simulink model "Ann_Pedals_SavePopup_newPwrCalib"  (Simulink 6.6)
settings: Solver=ode3  StartTime=0.0  StopTime=inf  RelTol=1e-3
StopFcn:
  | %% Name .mat file
  | 
  |     datime = datestr(now);
  |     colon = datime == ':';
  |     space = datime == ' ';
  |     dash  = datime == '-';
  |     datime(colon) = '';
  |     datime(space) = '_';
  |     datime(dash) = '';
  | 
  |     prompt = {'Subject #?','When? (PRE,POST,etc.)','Type of test? (forcepedals)', 'Loaded? (Enter loaded or unloaded)','Trial #? (1,2,...)'};
  | 
  |     dlgTitle = 'File Name';
  |     numlines = 1;
  |     default = {'000','PREPOST','forcepedals','loadedunloaded','1'};
  |     userinfo = inputdlg(prompt,dlgTitle,numlines,default);
  | 
  |     if isempty(userinfo) == 0
  |         sub = userinfo{1};
  |         reltime = userinfo{2};
  |         testype = userinfo{3};
  |         resist  = userinfo{4};
  |         trial   = userinfo{5};
  | 
  |         Filename = strcat('FESCycling_',sub,'_',reltime,'_',testype,'_',resist,'_',trial,'_',datime)
  | 
  | %     cd path_file
  | %
  |         save(Filename)
  |     end
values from neighbouring files (symbols this model uses):
  freq_range = 1022.16    [force_test_load.m]    (also in force_test_load_AnnSavePopup.m = 466.8; force_test_load_orig.m = 466.8; param.m = 865.41)
  freq_zero = -38.15    [force_test_load.m]    (also in force_test_load_AnnSavePopup.m = 116.7756; force_test_load_orig.m = 116.7756; param.m = 39.49)
  slope = 15.81    [force_test_load.m]    (also in force_test_load_AnnSavePopup.m = 14.1374; force_test_load_orig.m = 14.1374; param.m = 14.1374)
undefined symbols (not defined in the file or in its folder): analoginput, parameters
libraries: daqlib x1, ni_lib x1
settings Model: Creator=research  LastModifiedBy=research

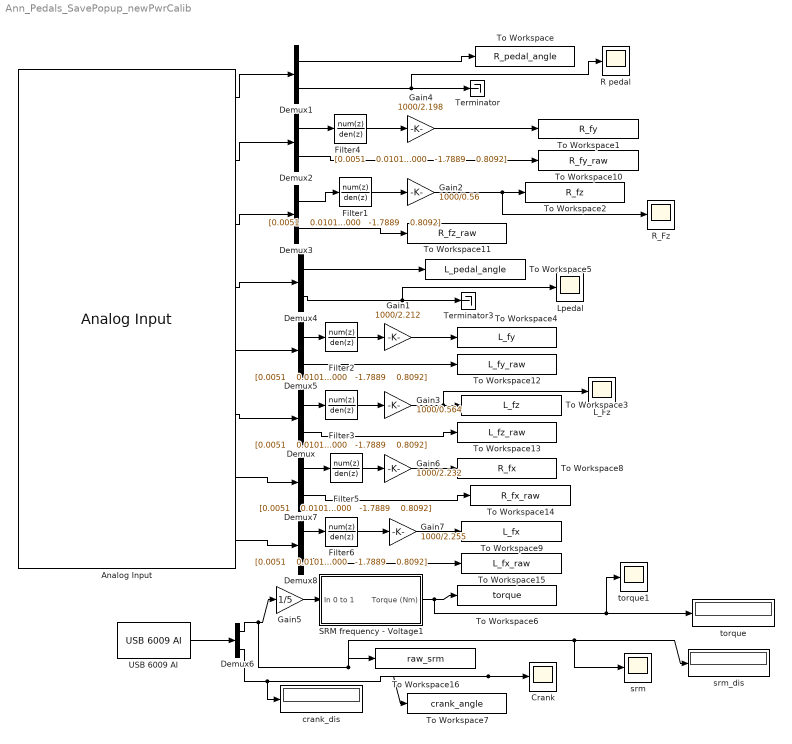
== system Ann_Pedals_SavePopup_newPwrCalib ==
  Analog Input : daqlib/Analog Input  DialogController=daqcreatedialog  DialogControllerArgs=DataTag0  AcqMode=0  Device=nidaq Dev1 (DAQCard-6062E)  ObjConstructor=analoginput('nidaq','Dev1')  SampleRate=1000  ActualRate=1000  SamplesPerFrame=2  InputType=Differential  NChannelsSelected=8  Channels=1$0$$1$#1$1$$11$#1$2$$11$#1$3$$1$#1$4$$11$#1$5$$11$#1$6$$11$#1$7$$11$#  NPorts=1 per hardware channel  DataType=double
      settings: SignalType=Sample-based
  Crank : Scope
      settings: YMin=0  YMax=5.25
  Demux{,1..8} (9 alike) : Demux  Outputs=2
  Filter{1..6} (6 alike) : DiscreteTransferFcn  Numerator="[0.0051    0.0101    0.0051]"  Denominator="[1.0000   -1.7889    0.8092]"  SampleTime=-1
  Gain1 : Gain  Gain=1000/2.212
  Gain2 : Gain  Gain=1000/0.56
  Gain3 : Gain  Gain=1000/0.564
  Gain4 : Gain  Gain=1000/2.198
  Gain5 : Gain  Gain=1/5
  Gain6 : Gain  Gain=1000/2.232
  Gain7 : Gain  Gain=1000/2.255
  L_Fz : Scope
      settings: YMin=-100  YMax=175  SaveName=ScopeData6
  Lpedal : Scope
      settings: YMin=0  YMax=10  SaveName=ScopeData3
  R pedal : Scope
      settings: YMin=0  YMax=9  SaveName=ScopeData5
  R_Fz : Scope
      settings: YMin=-75  YMax=150  SaveName=ScopeData2
  SRM frequency - Voltage1 : Subsystem
  Terminator : Terminator
  Terminator3 : Terminator
  To Workspace : ToWorkspace  VariableName=R_pedal_angle  SampleTime=-1  SaveFormat=Structure With Time
  To Workspace1 : ToWorkspace  VariableName=R_fy  SampleTime=-1  SaveFormat=Structure With Time
  To Workspace10 : ToWorkspace  VariableName=R_fy_raw  SampleTime=-1  SaveFormat=Structure With Time
  To Workspace11 : ToWorkspace  VariableName=R_fz_raw  SampleTime=-1  SaveFormat=Structure With Time
  To Workspace12 : ToWorkspace  VariableName=L_fy_raw  SampleTime=-1  SaveFormat=Structure With Time
  To Workspace13 : ToWorkspace  VariableName=L_fz_raw  SampleTime=-1  SaveFormat=Structure With Time
  To Workspace14 : ToWorkspace  VariableName=R_fx_raw  SampleTime=-1  SaveFormat=Structure With Time
  To Workspace15 : ToWorkspace  VariableName=L_fx_raw  SampleTime=-1  SaveFormat=Structure With Time
  To Workspace16 : ToWorkspace  VariableName=raw_srm  SampleTime=-1  SaveFormat=Structure With Time
  To Workspace2 : ToWorkspace  VariableName=R_fz  SampleTime=-1  SaveFormat=Structure With Time
  To Workspace3 : ToWorkspace  VariableName=L_fz  SampleTime=-1  SaveFormat=Structure With Time
  To Workspace4 : ToWorkspace  VariableName=L_fy  SampleTime=-1  SaveFormat=Structure With Time
  To Workspace5 : ToWorkspace  VariableName=L_pedal_angle  SampleTime=-1  SaveFormat=Structure With Time
  To Workspace6 : ToWorkspace  VariableName=torque  SampleTime=-1  SaveFormat=Structure With Time
  To Workspace7 : ToWorkspace  VariableName=crank_angle  SampleTime=-1  SaveFormat=Structure With Time
  To Workspace8 : ToWorkspace  VariableName=R_fx  SampleTime=-1  SaveFormat=Structure With Time
  To Workspace9 : ToWorkspace  VariableName=L_fx  SampleTime=-1  SaveFormat=Structure With Time
  USB 6009 AI : ni_lib/USB 6009 AI  channels=[1 3]  Ts=0.01  inp_min=-5  inp_max=5  terminalcfg=RSE
  crank_dis : Display
  srm : Scope
      settings: TimeRange=20  YMin=0  YMax=3.5
  srm_dis : Display
  torque : Display
  torque1 : Scope
      settings: TimeRange=20  YMin=-200  YMax=1100  SaveName=ScopeData7
  wires:
  Analog Input/1 -> Demux1/1
  Demux1/1 -> To Workspace/1
  Demux1/2 -> Terminator/1, R pedal/1
  Analog Input/2 -> Demux2/1
  Demux2/1 -> Filter4/1
  Demux/1 -> Filter3/1
  Analog Input/3 -> Demux3/1
  Analog Input/4 -> Demux4/1
  Demux4/1 -> To Workspace5/1
  Demux4/2 -> Lpedal/1, Terminator3/1
  Analog Input/5 -> Demux5/1
  Demux5/1 -> Filter2/1
  Analog Input/6 -> Demux/1
  Filter1/1 -> Gain2/1
  Demux3/1 -> Filter1/1
  Gain2/1 -> To Workspace2/1, R_Fz/1
  Filter3/1 -> Gain3/1
  Gain3/1 -> To Workspace3/1, L_Fz/1
  Filter2/1 -> Gain1/1
  Gain1/1 -> To Workspace4/1
  Filter4/1 -> Gain4/1
  Gain4/1 -> To Workspace1/1
  Gain5/1 -> SRM frequency - Voltage1/1(In 0 to 1)
  SRM frequency - Voltage1/1(Torque (Nm)) -> To Workspace6/1, torque/1, torque1/1
  USB 6009 AI/1 -> Demux6/1
  Demux6/1 -> Gain5/1, To Workspace16/1, srm/1, srm_dis/1
  Demux6/2 -> To Workspace7/1, Crank/1, crank_dis/1
  Analog Input/8 -> Demux8/1
  Analog Input/7 -> Demux7/1
  Demux7/1 -> Filter5/1
  Demux8/1 -> Filter6/1
  Filter5/1 -> Gain6/1
  Filter6/1 -> Gain7/1
  Gain6/1 -> To Workspace8/1
  Gain7/1 -> To Workspace9/1
  Demux2/2 -> To Workspace10/1
  Demux3/2 -> To Workspace11/1
  Demux5/2 -> To Workspace12/1
  Demux/2 -> To Workspace13/1
  Demux7/2 -> To Workspace14/1
  Demux8/2 -> To Workspace15/1

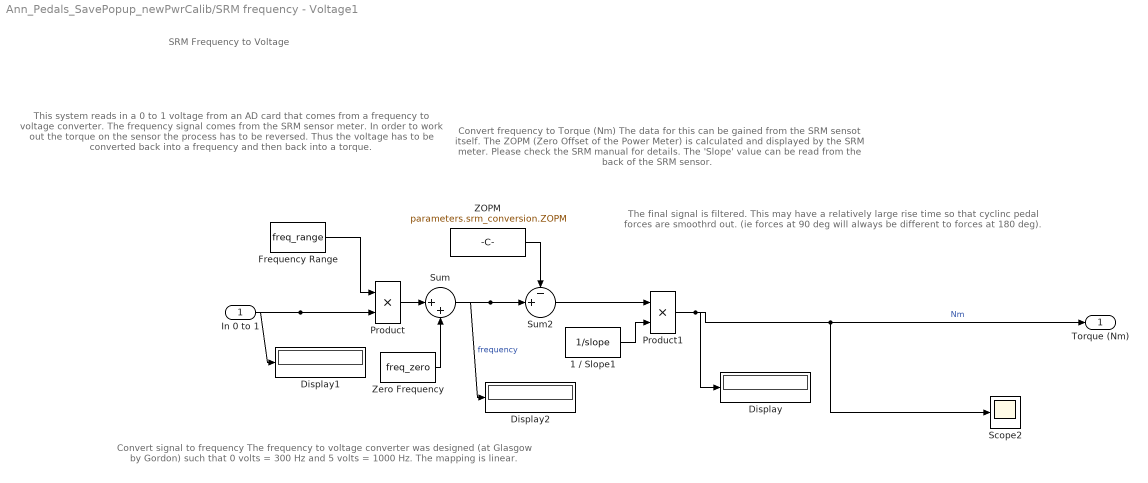
== system Ann_Pedals_SavePopup_newPwrCalib/SRM frequency - Voltage1 ==
  note: Convert frequency to Torque (Nm)
      |
      | The data for this can be gained
      | from the SRM sensot itself. The
      | ZOPM (Zero Offset of the Power
      | Meter) is calculated and displayed
      | by the SRM meter.  Please check
      | the SRM manual for details. The
      | 'Slope' value can be read from the
      | back of the SRM sensor.
  note: SRM Frequency to Voltage
  note: This system reads in a 0 to 1 voltage
      | from an AD card that comes from a
      | frequency to voltage converter.  The
      | frequency signal comes from the SRM
      | sensor meter.  In order to work out the
      | torque on the sensor the process has
      | to be reversed.  Thus the voltage has
      | to be converted back into a frequency
      | and then back into a torque.
  note: Convert signal to frequency
      |
      | The frequency to voltage converter
      | was designed (at Glasgow by
      | Gordon) such that 0 volts = 300 Hz
      | and 5 volts = 1000 Hz.  The
      | mapping is linear.
  note: The final signal is filtered.
      | This may have a relatively
      | large rise time so that
      | cyclinc pedal forces are
      | smoothrd out. (ie forces at
      | 90 deg will always be
      | different to forces at 180
      | deg).
  In 0 to 1 : Inport
  1 / Slope1 : Constant  Value=1/slope
  Display : Display
  Display1 : Display
  Display2 : Display
  Frequency Range : Constant  Value=freq_range
  Product : Product  SampleTime=0.01  SaturateOnIntegerOverflow=on  InputSameDT=on
  Product1 : Product  SampleTime=0.01  SaturateOnIntegerOverflow=on  InputSameDT=on
  Scope2 : Scope
      settings: YMin=-0.1  YMax=0.45  SaveName=ScopeData4
  Sum : Sum  Inputs=|++  SampleTime=0.01  SaturateOnIntegerOverflow=on  InputSameDT=on
  Sum2 : Sum  Inputs=-+|  SampleTime=0.01  SaturateOnIntegerOverflow=on  InputSameDT=on
  ZOPM : Constant  Value=parameters.srm_conversion.ZOPM
  Zero Frequency : Constant  Value=freq_zero
  Torque (Nm) : Outport
  wires:
  Zero Frequency/1 -> Sum/2
  1 / Slope1/1 -> Product1/2
  ZOPM/1 -> Sum2/1
  Frequency Range/1 -> Product/1
  Sum/1 -> Sum2/2, Display2/1  "frequency"
  In 0 to 1/1 -> Product/2, Display1/1
  Product/1 -> Sum/1
  Sum2/1 -> Product1/1
  Product1/1 -> Scope2/1, Torque (Nm)/1, Display/1  "Nm"
